simulink subsystem "pDMP"  (R2020a)
settings: Solver=VariableStepAuto  StartTime=0.0  StopTime=10.0  RelTol=1e-3
PreLoadFcn:
  | addpath(genpath(pwd));
settings Model: Creator=12927  LastModifiedBy=12927

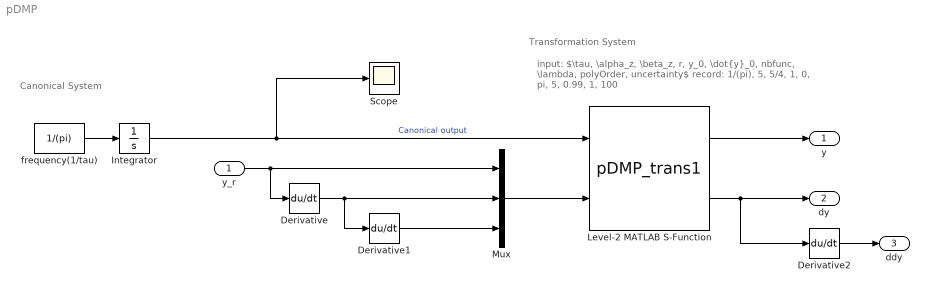
== system pDMP ==
  note: Canonical System
  note: Transformation System
  note: input: $\tau, \alpha_z, \beta_z, r, y_0, \dot{y}_0, nbfunc, \lambda, polyOrder, uncertainty$
      |
      | record: 1/(pi), 5, 5/4, 1, 0, pi, 5, 0.99, 1, 100
  y_r : Inport
  Derivative : Derivative
  Derivative1 : Derivative
  Derivative2 : Derivative
  Integrator : Integrator
  Level-2 MATLAB S-Function : M-S-Function  FunctionName=pDMP_trans1  Parameters=1/(pi), 5, 5/4, 1, 0, pi, 5, 0.99, 1, 100
  Mux : Mux  Inputs=3
  Scope : Scope
  frequency(1/tau) : Constant  Value=1/(pi)
  y : Outport
  dy : Outport  Port=2
  ddy : Outport  Port=3
  wires:
  Integrator/1 -> Level-2 MATLAB S-Function/1, Scope/1  "Canonical output"
  y_r/1 -> Derivative/1, Mux/1
  Derivative/1 -> Derivative1/1, Mux/2
  Derivative1/1 -> Mux/3
  Level-2 MATLAB S-Function/1 -> y/1
  Level-2 MATLAB S-Function/2 -> dy/1, Derivative2/1
  Mux/1 -> Level-2 MATLAB S-Function/2
  frequency(1/tau)/1 -> Integrator/1
  Derivative2/1 -> ddy/1
